simulink model "SP_OEL"  (R2023b)
settings: Solver=VariableStepAuto  StartTime=0.0  StopTime=1  RelTol=1e-3
undefined symbols (not defined in the file or in its folder): relay1, relay2, source
libraries: ee_lib x31, fl_lib x16, eeGeneralControl x8, nesl_utility x7, simulink x4, simulink_extras x4, spspowerguiLib x1
(part 2 of 2)

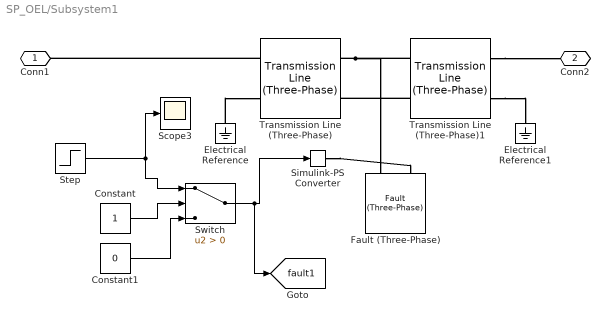
== system SP_OEL/Subsystem1 ==
  Constant : Constant
  Constant1 : Constant  Value=0
  Electrical Reference : fl_lib/Electrical/Electrical Elements/Electrical Reference
  Electrical Reference1 : fl_lib/Electrical/Electrical Elements/Electrical Reference
  Fault (Three-Phase) : ee_lib/Utilities/Fault (Three-Phase)  fault_type_option=1  R_pn_fault=1e-6 Ohm  R_ng_fault=1e-6 Ohm  exposemeasurement=ee.enum.exposemeasurement.hidden  enable_external_fault=ee.enum.external_fault.visible  fault_threshold=0.5  fault_condition=1  fault_resettable=1  enable_temporal_fault=0  fault_start_time=1 s  fault_duration=0.1 s  G_parasitic=1e-6 1/Ohm
      settings: InternalSimscapePortConfiguration="{\"Bottom\":[],\"Left\":[{\"id\":\"N\",\"label\":\"~\",\"type\":\"foundation.electrical.three_phase\"},{\"id\":\"F\",\"label\":\"F\",\"type\":\"input\"}],\"Right\":[],\"Top\":[]}"
  Scope3 : Scope
  Simulink-PS Converter : nesl_utility/Simulink-PS Converter  PhysicalDomain=network_engine_domain  SubClassName=ps_input  LeftPortType=input  RightPortType=output  PseudoPeriodic=off  Frequencies=[]  NoiseDistribution=none  NoiseParameters=[]  Unit=1  AffineConversion=off  FilteringAndDerivatives=provide  SimscapeFilterOrder=1  InputFilterTimeConstant=0.001  UdotUserProvided=0
  Step : Step  Time=0  After=0  SampleTime=0
  Switch : Switch  Criteria=u2 > Threshold  SaturateOnIntegerOverflow=off  InputSameDT=off
  Transmission Line (Three-Phase) : ee_lib/Passive/Lines/Transmission Line (Three-Phase)  length=1 km  freq=50 Hz  R=0.0268 Ohm/km  L=0.32 mH/km  M=0.0 mH/km  Cl=0.37 uF/km  Cg=0.1 uF/km  Rm=0 Ohm/km  ModelTwoSections=ee.enum.enable.no  N=1  InterfacePosition=0.5 km  N1sec=1  N2sec=1  Access_ground=ee.enum.enable.no  R_parasitic=1e-4 Ohm  G_parasitic=1e-4 1/Ohm  EnableFault=false  fault_type_option=ee.enum.fault_type_option.ag  R_pn_fault=1e-3 Ohm  R_ng_fault=1e-3 Ohm  unfaulted_G_parasitic=1e-6 1/Ohm
      settings: InternalSimscapePortConfiguration="{\"Bottom\":[],\"Left\":[{\"id\":\"N1\",\"label\":\"~1\",\"type\":\"foundation.electrical.three_phase\"},{\"id\":\"g1\",\"label\":\"g1\",\"type\":\"foundation.electrical.electrical\"}],\"Right\":[{\"id\":\"N2\",\"label\":\"~2\",\"type\":\"foundation.electrical.three_phase\"},{\"id\":\"g2\",\"label\":\"g2\",\"type\":\"foundation.electrical.electrical\"}],\"Top\":[]}"
  Transmission Line (Three-Phase)1 : ee_lib/Passive/Lines/Transmission Line (Three-Phase)  length=9 km  freq=50 Hz  R=0.0268 Ohm/km  L=0.32 mH/km  M=0.0 mH/km  Cl=0.37 uF/km  Cg=0.1 uF/km  Rm=0 Ohm/km  ModelTwoSections=ee.enum.enable.no  N=1  InterfacePosition=0.5 km  N1sec=1  N2sec=1  Access_ground=ee.enum.enable.no  R_parasitic=1e-4 Ohm  G_parasitic=1e-4 1/Ohm  EnableFault=false  fault_type_option=ee.enum.fault_type_option.ag  R_pn_fault=1e-3 Ohm  R_ng_fault=1e-3 Ohm  unfaulted_G_parasitic=1e-6 1/Ohm
      settings: InternalSimscapePortConfiguration="{\"Bottom\":[],\"Left\":[{\"id\":\"N1\",\"label\":\"~1\",\"type\":\"foundation.electrical.three_phase\"},{\"id\":\"g1\",\"label\":\"g1\",\"type\":\"foundation.electrical.electrical\"}],\"Right\":[{\"id\":\"N2\",\"label\":\"~2\",\"type\":\"foundation.electrical.three_phase\"},{\"id\":\"g2\",\"label\":\"g2\",\"type\":\"foundation.electrical.electrical\"}],\"Top\":[]}"
  Conn1 : PMIOPort  Side=Left
  Conn2 : PMIOPort  Port=2  Side=Right
  tag scope: fault1=global
  wires:
  Switch/1 -> [fault1], Simulink-PS Converter/1
  Constant1/1 -> Switch/3
  Constant/1 -> Switch/2
  Step/1 -> Scope3/1, Switch/1
  connections:
  Transmission Line (Three-Phase)1/RConn2 -- Electrical Reference1/LConn1
  Electrical Reference/LConn1 -- Transmission Line (Three-Phase)/LConn2
  Simulink-PS Converter/RConn1 -- Fault (Three-Phase)/LConn2
  Transmission Line (Three-Phase)1/RConn1 -- Conn2/RConn1
  Transmission Line (Three-Phase)/RConn1 -- Transmission Line (Three-Phase)1/LConn1 -- Fault (Three-Phase)/LConn1
  Transmission Line (Three-Phase)/LConn1 -- Conn1/RConn1
  Transmission Line (Three-Phase)1/LConn2 -- Transmission Line (Three-Phase)/RConn2

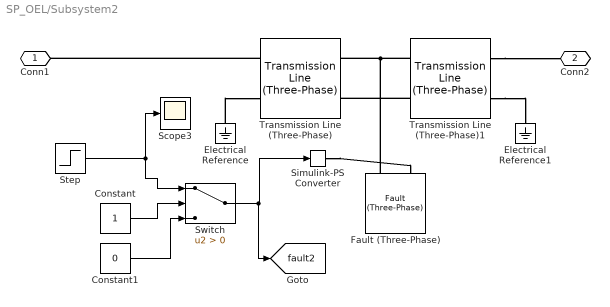
== system SP_OEL/Subsystem2 ==
  Constant : Constant
  Constant1 : Constant  Value=0
  Electrical Reference : fl_lib/Electrical/Electrical Elements/Electrical Reference
  Electrical Reference1 : fl_lib/Electrical/Electrical Elements/Electrical Reference
  Fault (Three-Phase) : ee_lib/Utilities/Fault (Three-Phase)  fault_type_option=1  R_pn_fault=1e-6 Ohm  R_ng_fault=1e-6 Ohm  exposemeasurement=ee.enum.exposemeasurement.hidden  enable_external_fault=ee.enum.external_fault.visible  fault_threshold=0.5  fault_condition=1  fault_resettable=1  enable_temporal_fault=0  fault_start_time=1 s  fault_duration=0.1 s  G_parasitic=1e-6 1/Ohm
      settings: InternalSimscapePortConfiguration="{\"Bottom\":[],\"Left\":[{\"id\":\"N\",\"label\":\"~\",\"type\":\"foundation.electrical.three_phase\"},{\"id\":\"F\",\"label\":\"F\",\"type\":\"input\"}],\"Right\":[],\"Top\":[]}"
  Scope3 : Scope
  Simulink-PS Converter : nesl_utility/Simulink-PS Converter  PhysicalDomain=network_engine_domain  SubClassName=ps_input  LeftPortType=input  RightPortType=output  PseudoPeriodic=off  Frequencies=[]  NoiseDistribution=none  NoiseParameters=[]  Unit=1  AffineConversion=off  FilteringAndDerivatives=provide  SimscapeFilterOrder=1  InputFilterTimeConstant=0.001  UdotUserProvided=0
  Step : Step  Time=0.2  SampleTime=0
  Switch : Switch  Criteria=u2 > Threshold  SaturateOnIntegerOverflow=off  InputSameDT=off
  Transmission Line (Three-Phase) : ee_lib/Passive/Lines/Transmission Line (Three-Phase)  length=1 km  freq=50 Hz  R=0.0268 Ohm/km  L=0.32 mH/km  M=0.0 mH/km  Cl=0.37 uF/km  Cg=0.1 uF/km  Rm=0 Ohm/km  ModelTwoSections=ee.enum.enable.no  N=1  InterfacePosition=0.5 km  N1sec=1  N2sec=1  Access_ground=ee.enum.enable.no  R_parasitic=1e-4 Ohm  G_parasitic=1e-4 1/Ohm  EnableFault=false  fault_type_option=ee.enum.fault_type_option.ag  R_pn_fault=1e-3 Ohm  R_ng_fault=1e-3 Ohm  unfaulted_G_parasitic=1e-6 1/Ohm
      settings: InternalSimscapePortConfiguration="{\"Bottom\":[],\"Left\":[{\"id\":\"N1\",\"label\":\"~1\",\"type\":\"foundation.electrical.three_phase\"},{\"id\":\"g1\",\"label\":\"g1\",\"type\":\"foundation.electrical.electrical\"}],\"Right\":[{\"id\":\"N2\",\"label\":\"~2\",\"type\":\"foundation.electrical.three_phase\"},{\"id\":\"g2\",\"label\":\"g2\",\"type\":\"foundation.electrical.electrical\"}],\"Top\":[]}"
  Transmission Line (Three-Phase)1 : ee_lib/Passive/Lines/Transmission Line (Three-Phase)  length=9 km  freq=50 Hz  R=0.0268 Ohm/km  L=0.32 mH/km  M=0.0 mH/km  Cl=0.37 uF/km  Cg=0.1 uF/km  Rm=0 Ohm/km  ModelTwoSections=ee.enum.enable.no  N=1  InterfacePosition=0.5 km  N1sec=1  N2sec=1  Access_ground=ee.enum.enable.no  R_parasitic=1e-4 Ohm  G_parasitic=1e-4 1/Ohm  EnableFault=false  fault_type_option=ee.enum.fault_type_option.ag  R_pn_fault=1e-3 Ohm  R_ng_fault=1e-3 Ohm  unfaulted_G_parasitic=1e-6 1/Ohm
      settings: InternalSimscapePortConfiguration="{\"Bottom\":[],\"Left\":[{\"id\":\"N1\",\"label\":\"~1\",\"type\":\"foundation.electrical.three_phase\"},{\"id\":\"g1\",\"label\":\"g1\",\"type\":\"foundation.electrical.electrical\"}],\"Right\":[{\"id\":\"N2\",\"label\":\"~2\",\"type\":\"foundation.electrical.three_phase\"},{\"id\":\"g2\",\"label\":\"g2\",\"type\":\"foundation.electrical.electrical\"}],\"Top\":[]}"
  Conn1 : PMIOPort  Side=Left
  Conn2 : PMIOPort  Port=2  Side=Right
  tag scope: fault2=global
  wires:
  Step/1 -> Switch/1, Scope3/1
  Constant/1 -> Switch/2
  Constant1/1 -> Switch/3
  Switch/1 -> [fault2], Simulink-PS Converter/1
  connections:
  Transmission Line (Three-Phase)1/LConn2 -- Transmission Line (Three-Phase)/RConn2
  Transmission Line (Three-Phase)/LConn1 -- Conn1/RConn1
  Transmission Line (Three-Phase)1/LConn1 -- Fault (Three-Phase)/LConn1 -- Transmission Line (Three-Phase)/RConn1
  Transmission Line (Three-Phase)1/RConn1 -- Conn2/RConn1
  Simulink-PS Converter/RConn1 -- Fault (Three-Phase)/LConn2
  Electrical Reference/LConn1 -- Transmission Line (Three-Phase)/LConn2
  Transmission Line (Three-Phase)1/RConn2 -- Electrical Reference1/LConn1

== system SP_OEL/ Sensor1/Sensor dynamics ==
  V : Inport
  Demux : Demux  Outputs=3
  Mux : Mux  Inputs=3
  Transfer Fcn : TransferFcn  Denominator=[relay1.sampleTime 1]
  Transfer Fcn1 : TransferFcn  Denominator=[relay1.sampleTime 1]
  Transfer Fcn2 : TransferFcn  Denominator=[relay1.sampleTime 1]
  I : Outport
  wires:
  Transfer Fcn/1 -> Mux/1
  Demux/1 -> Transfer Fcn/1
  Demux/3 -> Transfer Fcn2/1
  Mux/1 -> I/1
  Transfer Fcn2/1 -> Mux/3
  Transfer Fcn1/1 -> Mux/2
  Demux/2 -> Transfer Fcn1/1
  V/1 -> Demux/1

== system SP_OEL/ Sensor2/Sensor dynamics ==
  V : Inport
  Demux : Demux  Outputs=3
  Mux : Mux  Inputs=3
  Transfer Fcn : TransferFcn  Denominator=[relay2.sampleTime 1]
  Transfer Fcn1 : TransferFcn  Denominator=[relay2.sampleTime 1]
  Transfer Fcn2 : TransferFcn  Denominator=[relay2.sampleTime 1]
  I : Outport
  wires:
  Transfer Fcn/1 -> Mux/1
  Demux/1 -> Transfer Fcn/1
  Demux/3 -> Transfer Fcn2/1
  Mux/1 -> I/1
  Transfer Fcn2/1 -> Mux/3
  Transfer Fcn1/1 -> Mux/2
  Demux/2 -> Transfer Fcn1/1
  V/1 -> Demux/1

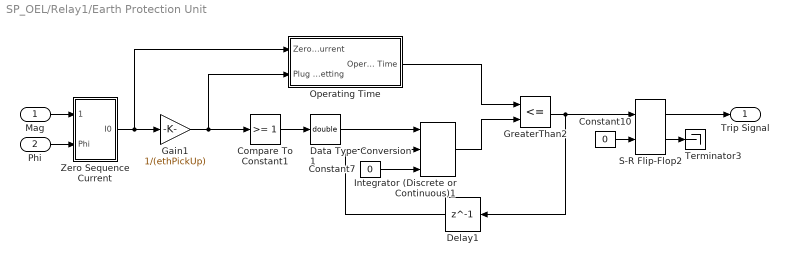
== system SP_OEL/Relay1/Earth Protection Unit ==
  Mag : Inport
  Phi : Inport  Port=2
  Compare To Constant1 : simulink/Logic and Bit Operations/Compare To Constant  relop=>=  const=1  OutDataTypeStr=boolean
  Constant10 : Constant  Value=0  OutDataTypeStr=boolean
  Constant7 : Constant  Value=0  OutDataTypeStr=double
  Data Type Conversion1 : DataTypeConversion  OutDataTypeStr=double  SaturateOnIntegerOverflow=off  RndMeth=Floor
  Delay1 : Delay  DelayLength=1
  Gain1 : Gain  Gain=1/(ethPickUp)
  GreaterThan2 : RelationalOperator  Operator=<=  OutDataTypeStr=boolean  RndMeth=Simplest  InputSameDT=off
  Integrator (Discrete or Continuous)1 : eeGeneralControl/Integrator (Discrete or Continuous)  LabelModeActiveChoice=Discrete  ExternalReset=falling  LimitType=Anti-windup  B=inf  A=-inf  Ts=sampleTime
  Operating Time : Subsystem
  S-R Flip-Flop2 : simulink_extras/Flip Flops/S-R Flip-Flop  initial_condition=0
  Terminator3 : Terminator
  Zero Sequence Current : Subsystem
  Trip Signal : Outport
  wires:
  Gain1/1 -> Operating Time/2(Plug Setting), Compare To Constant1/1
  Compare To Constant1/1 -> Data Type Conversion1/1
  GreaterThan2/1 -> Delay1/1, S-R Flip-Flop2/1
  Delay1/1 -> Integrator (Discrete or Continuous)1/2
  Constant10/1 -> S-R Flip-Flop2/2
  Zero Sequence Current/1(I0) -> Gain1/1, Operating Time/1(Zero Sequence Current)
  Data Type Conversion1/1 -> Integrator (Discrete or Continuous)1/1
  Integrator (Discrete or Continuous)1/1 -> GreaterThan2/2
  Operating Time/1(Operating Time) -> GreaterThan2/1
  S-R Flip-Flop2/2 -> Terminator3/1
  Constant7/1 -> Integrator (Discrete or Continuous)1/3
  Phi/1 -> Zero Sequence Current/2(Phi)
  Mag/1 -> Zero Sequence Current/1(Mag)
  S-R Flip-Flop2/1 -> Trip Signal/1

== system SP_OEL/Relay1/Fourier Analysis ==
  Current : Inport
  Add1 : Sum  Inputs=-+
  Delay3 : Delay  DelayLength=1
  Fourier Analysis2 : eeGeneralControl/Fourier Analysis  f=ratedFrequency  n=[1]  M0=0  Ph0=0  BufferSize=8192  Ts=sampleTime
  Gain : Gain  Gain=1/sqrt(2)
  Moving Average : eeGeneralControl/Moving Average  VariantControl=Variant1  LabelModeActiveChoice=Discrete  f=50  x0=0  BufferSize=8192  Ts=sampleTime
  Magnitude : Outport
  Angle : Outport  Port=2
  wires:
  Delay3/1 -> Add1/2, Moving Average/1
  Current/1 -> Delay3/1
  Fourier Analysis2/2 -> Angle/1
  Moving Average/1 -> Add1/1
  Add1/1 -> Fourier Analysis2/1
  Fourier Analysis2/1 -> Gain/1
  Gain/1 -> Magnitude/1

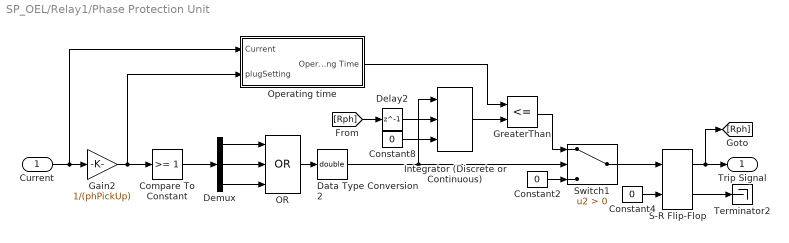
== system SP_OEL/Relay1/Phase Protection Unit ==
  Current : Inport
  Compare To Constant : simulink/Logic and Bit Operations/Compare To Constant  relop=>=  const=1  OutDataTypeStr=boolean
  Constant2 : Constant  Value=0  OutDataTypeStr=boolean
  Constant4 : Constant  Value=0  OutDataTypeStr=boolean
  Constant8 : Constant  Value=0  OutDataTypeStr=double
  Data Type Conversion2 : DataTypeConversion  OutDataTypeStr=double  SaturateOnIntegerOverflow=off  RndMeth=Floor
  Delay2 : Delay  DelayLength=1
  Demux : Demux  Outputs=3
  Gain2 : Gain  Gain=1/(phPickUp)
  GreaterThan : RelationalOperator  Operator=<=  OutDataTypeStr=boolean  RndMeth=Simplest  InputSameDT=off
  Integrator (Discrete or Continuous) : eeGeneralControl/Integrator (Discrete or Continuous)  LabelModeActiveChoice=Discrete  ExternalReset=falling  LimitType=Anti-windup  B=inf  A=-inf  Ts=sampleTime
  OR : Logic  Operator=OR  Inputs=3  IconShape=distinctive  AllPortsSameDT=off  OutDataTypeStr=boolean
  "Operating time " : Subsystem
  S-R Flip-Flop : simulink_extras/Flip Flops/S-R Flip-Flop  initial_condition=0
  Switch1 : Switch  Criteria=u2 > Threshold  OutDataTypeStr=boolean  SaturateOnIntegerOverflow=off  InputSameDT=off
  Terminator2 : Terminator
  Trip Signal : Outport
  wires:
  Data Type Conversion2/1 -> Integrator (Discrete or Continuous)/1, Switch1/2
  Gain2/1 -> "Operating time "/2(plugSetting), Compare To Constant/1
  Constant2/1 -> Switch1/3
  Demux/2 -> OR/2
  OR/1 -> Data Type Conversion2/1
  Integrator (Discrete or Continuous)/1 -> GreaterThan/2
  Demux/3 -> OR/3
  Current/1 -> Gain2/1, "Operating time "/1(Current)
  GreaterThan/1 -> Switch1/1
  "Operating time "/1(Operating Time) -> GreaterThan/1
  Constant4/1 -> S-R Flip-Flop/2
  S-R Flip-Flop/2 -> Terminator2/1
  Switch1/1 -> S-R Flip-Flop/1
  Demux/1 -> OR/1
  Constant8/1 -> Integrator (Discrete or Continuous)/3
  Compare To Constant/1 -> Demux/1
  S-R Flip-Flop/1 -> Trip Signal/1, [Rph]
  Delay2/1 -> Integrator (Discrete or Continuous)/2
  [Rph] -> Delay2/1

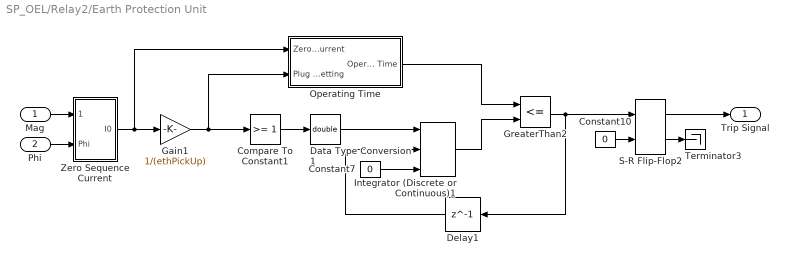
== system SP_OEL/Relay2/Earth Protection Unit ==
  Mag : Inport
  Phi : Inport  Port=2
  Compare To Constant1 : simulink/Logic and Bit Operations/Compare To Constant  relop=>=  const=1  OutDataTypeStr=boolean
  Constant10 : Constant  Value=0  OutDataTypeStr=boolean
  Constant7 : Constant  Value=0  OutDataTypeStr=double
  Data Type Conversion1 : DataTypeConversion  OutDataTypeStr=double  SaturateOnIntegerOverflow=off  RndMeth=Floor
  Delay1 : Delay  DelayLength=1
  Gain1 : Gain  Gain=1/(ethPickUp)
  GreaterThan2 : RelationalOperator  Operator=<=  OutDataTypeStr=boolean  RndMeth=Simplest  InputSameDT=off
  Integrator (Discrete or Continuous)1 : eeGeneralControl/Integrator (Discrete or Continuous)  LabelModeActiveChoice=Discrete  ExternalReset=falling  LimitType=Anti-windup  B=inf  A=-inf  Ts=sampleTime
  Operating Time : Subsystem
  S-R Flip-Flop2 : simulink_extras/Flip Flops/S-R Flip-Flop  initial_condition=0
  Terminator3 : Terminator
  Zero Sequence Current : Subsystem
  Trip Signal : Outport
  wires:
  Gain1/1 -> Operating Time/2(Plug Setting), Compare To Constant1/1
  Compare To Constant1/1 -> Data Type Conversion1/1
  GreaterThan2/1 -> Delay1/1, S-R Flip-Flop2/1
  Delay1/1 -> Integrator (Discrete or Continuous)1/2
  Constant10/1 -> S-R Flip-Flop2/2
  Zero Sequence Current/1(I0) -> Gain1/1, Operating Time/1(Zero Sequence Current)
  Data Type Conversion1/1 -> Integrator (Discrete or Continuous)1/1
  Integrator (Discrete or Continuous)1/1 -> GreaterThan2/2
  Operating Time/1(Operating Time) -> GreaterThan2/1
  S-R Flip-Flop2/2 -> Terminator3/1
  Constant7/1 -> Integrator (Discrete or Continuous)1/3
  Phi/1 -> Zero Sequence Current/2(Phi)
  Mag/1 -> Zero Sequence Current/1(Mag)
  S-R Flip-Flop2/1 -> Trip Signal/1

== system SP_OEL/Relay2/Fourier Analysis ==
  Current : Inport
  Add1 : Sum  Inputs=-+
  Delay3 : Delay  DelayLength=1
  Fourier Analysis2 : eeGeneralControl/Fourier Analysis  f=ratedFrequency  n=[1]  M0=0  Ph0=0  BufferSize=8192  Ts=sampleTime
  Gain : Gain  Gain=1/sqrt(2)
  Moving Average : eeGeneralControl/Moving Average  VariantControl=Variant1  LabelModeActiveChoice=Discrete  f=50  x0=0  BufferSize=8192  Ts=sampleTime
  Magnitude : Outport
  Angle : Outport  Port=2
  wires:
  Delay3/1 -> Add1/2, Moving Average/1
  Current/1 -> Delay3/1
  Fourier Analysis2/2 -> Angle/1
  Moving Average/1 -> Add1/1
  Add1/1 -> Fourier Analysis2/1
  Fourier Analysis2/1 -> Gain/1
  Gain/1 -> Magnitude/1

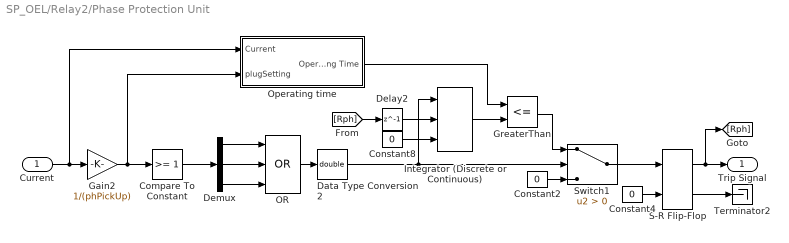
== system SP_OEL/Relay2/Phase Protection Unit ==
  Current : Inport
  Compare To Constant : simulink/Logic and Bit Operations/Compare To Constant  relop=>=  const=1  OutDataTypeStr=boolean
  Constant2 : Constant  Value=0  OutDataTypeStr=boolean
  Constant4 : Constant  Value=0  OutDataTypeStr=boolean
  Constant8 : Constant  Value=0  OutDataTypeStr=double
  Data Type Conversion2 : DataTypeConversion  OutDataTypeStr=double  SaturateOnIntegerOverflow=off  RndMeth=Floor
  Delay2 : Delay  DelayLength=1
  Demux : Demux  Outputs=3
  Gain2 : Gain  Gain=1/(phPickUp)
  GreaterThan : RelationalOperator  Operator=<=  OutDataTypeStr=boolean  RndMeth=Simplest  InputSameDT=off
  Integrator (Discrete or Continuous) : eeGeneralControl/Integrator (Discrete or Continuous)  LabelModeActiveChoice=Discrete  ExternalReset=falling  LimitType=Anti-windup  B=inf  A=-inf  Ts=sampleTime
  OR : Logic  Operator=OR  Inputs=3  IconShape=distinctive  AllPortsSameDT=off  OutDataTypeStr=boolean
  "Operating time " : Subsystem
  S-R Flip-Flop : simulink_extras/Flip Flops/S-R Flip-Flop  initial_condition=0
  Switch1 : Switch  Criteria=u2 > Threshold  OutDataTypeStr=boolean  SaturateOnIntegerOverflow=off  InputSameDT=off
  Terminator2 : Terminator
  Trip Signal : Outport
  wires:
  Data Type Conversion2/1 -> Integrator (Discrete or Continuous)/1, Switch1/2
  Gain2/1 -> "Operating time "/2(plugSetting), Compare To Constant/1
  Constant2/1 -> Switch1/3
  Demux/2 -> OR/2
  OR/1 -> Data Type Conversion2/1
  Integrator (Discrete or Continuous)/1 -> GreaterThan/2
  Demux/3 -> OR/3
  Current/1 -> Gain2/1, "Operating time "/1(Current)
  GreaterThan/1 -> Switch1/1
  "Operating time "/1(Operating Time) -> GreaterThan/1
  Constant4/1 -> S-R Flip-Flop/2
  S-R Flip-Flop/2 -> Terminator2/1
  Switch1/1 -> S-R Flip-Flop/1
  Demux/1 -> OR/1
  Constant8/1 -> Integrator (Discrete or Continuous)/3
  Compare To Constant/1 -> Demux/1
  S-R Flip-Flop/1 -> Trip Signal/1, [Rph]
  Delay2/1 -> Integrator (Discrete or Continuous)/2
  [Rph] -> Delay2/1

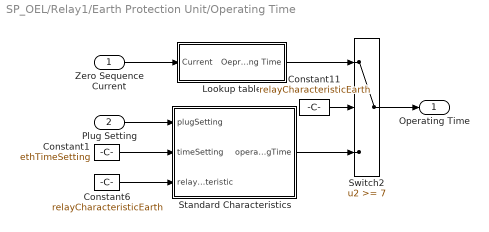
== system SP_OEL/Relay1/Earth Protection Unit/Operating Time ==
  Zero Sequence Current : Inport
  Plug Setting : Inport  Port=2
  Constant1 : Constant  Value=ethTimeSetting
  Constant11 : Constant  Value=relayCharacteristicEarth
  Constant6 : Constant  Value=relayCharacteristicEarth
  Lookup table : Subsystem
  Standard Characteristics : MATLAB Function  TreatAsAtomicUnit=on
  Switch2 : Switch  Threshold=7  SaturateOnIntegerOverflow=off  InputSameDT=off
  Operating Time : Outport
  wires:
  Constant1/1 -> Standard Characteristics/2(timeSetting)
  Lookup table/1(Oeprating Time) -> Switch2/1
  Constant6/1 -> Standard Characteristics/3(relayCharacteristic)
  Plug Setting/1 -> Standard Characteristics/1(plugSetting)
  Standard Characteristics/1(operatingTime) -> Switch2/3
  Constant11/1 -> Switch2/2
  Switch2/1 -> Operating Time/1
  Zero Sequence Current/1 -> Lookup table/1(Current)

== system SP_OEL/Relay1/Earth Protection Unit/Zero Sequence Current ==
  Mag : Inport
  Phi : Inport  Port=2
  Add : Sum  Inputs=+++
  Complex to Magnitude-Angle : ComplexToMagnitudeAngle  Output=Magnitude
  Demux1 : Demux  Outputs=3
  Gain : Gain  Gain=1/3
  Magnitude-Angle to Complex : MagnitudeAngleToComplex
  I0 : Outport
  wires:
  Demux1/2 -> Add/2
  Demux1/3 -> Add/3
  Phi/1 -> Magnitude-Angle to Complex/2
  Complex to Magnitude-Angle/1 -> Gain/1
  Demux1/1 -> Add/1
  Mag/1 -> Magnitude-Angle to Complex/1
  Magnitude-Angle to Complex/1 -> Demux1/1
  Add/1 -> Complex to Magnitude-Angle/1
  Gain/1 -> I0/1

== system SP_OEL/Relay1/Phase Protection Unit/Operating time  ==
  Current : Inport
  plugSetting : Inport  Port=2
  Constant : Constant  Value=phTimeSetting  VectorParams1D=off
  Constant3 : Constant  Value=relayCharacteristicPhase
  Constant9 : Constant  Value=relayCharacteristicPhase
  "Lookup table " : Subsystem
  MATLAB Function : MATLAB Function  TreatAsAtomicUnit=on
  Switch : Switch  Threshold=7  SaturateOnIntegerOverflow=off  InputSameDT=off
  Operating Time : Outport
  wires:
  Switch/1 -> Operating Time/1
  plugSetting/1 -> MATLAB Function/1(plugSetting)
  Constant9/1 -> Switch/2
  Constant/1 -> MATLAB Function/2(timeSetting)
  Constant3/1 -> MATLAB Function/3(relayCharacteristic)
  MATLAB Function/1(operatingTime) -> Switch/3
  "Lookup table "/1(Operating Time) -> Switch/1
  Current/1 -> "Lookup table "/1(Current)

== system SP_OEL/Relay2/Earth Protection Unit/Operating Time ==
  Zero Sequence Current : Inport
  Plug Setting : Inport  Port=2
  Constant1 : Constant  Value=ethTimeSetting
  Constant11 : Constant  Value=relayCharacteristicEarth
  Constant6 : Constant  Value=relayCharacteristicEarth
  Lookup table : Subsystem
  Standard Characteristics : MATLAB Function  TreatAsAtomicUnit=on
  Switch2 : Switch  Threshold=7  SaturateOnIntegerOverflow=off  InputSameDT=off
  Operating Time : Outport
  wires:
  Constant1/1 -> Standard Characteristics/2(timeSetting)
  Lookup table/1(Oeprating Time) -> Switch2/1
  Constant6/1 -> Standard Characteristics/3(relayCharacteristic)
  Plug Setting/1 -> Standard Characteristics/1(plugSetting)
  Standard Characteristics/1(operatingTime) -> Switch2/3
  Constant11/1 -> Switch2/2
  Switch2/1 -> Operating Time/1
  Zero Sequence Current/1 -> Lookup table/1(Current)

== system SP_OEL/Relay2/Earth Protection Unit/Zero Sequence Current ==
  Mag : Inport
  Phi : Inport  Port=2
  Add : Sum  Inputs=+++
  Complex to Magnitude-Angle : ComplexToMagnitudeAngle  Output=Magnitude
  Demux1 : Demux  Outputs=3
  Gain : Gain  Gain=1/3
  Magnitude-Angle to Complex : MagnitudeAngleToComplex
  I0 : Outport
  wires:
  Demux1/2 -> Add/2
  Demux1/3 -> Add/3
  Phi/1 -> Magnitude-Angle to Complex/2
  Complex to Magnitude-Angle/1 -> Gain/1
  Demux1/1 -> Add/1
  Mag/1 -> Magnitude-Angle to Complex/1
  Magnitude-Angle to Complex/1 -> Demux1/1
  Add/1 -> Complex to Magnitude-Angle/1
  Gain/1 -> I0/1

== system SP_OEL/Relay2/Phase Protection Unit/Operating time  ==
  Current : Inport
  plugSetting : Inport  Port=2
  Constant : Constant  Value=phTimeSetting  VectorParams1D=off
  Constant3 : Constant  Value=relayCharacteristicPhase
  Constant9 : Constant  Value=relayCharacteristicPhase
  "Lookup table " : Subsystem
  MATLAB Function : MATLAB Function  TreatAsAtomicUnit=on
  Switch : Switch  Threshold=7  SaturateOnIntegerOverflow=off  InputSameDT=off
  Operating Time : Outport
  wires:
  Switch/1 -> Operating Time/1
  plugSetting/1 -> MATLAB Function/1(plugSetting)
  Constant9/1 -> Switch/2
  Constant/1 -> MATLAB Function/2(timeSetting)
  Constant3/1 -> MATLAB Function/3(relayCharacteristic)
  MATLAB Function/1(operatingTime) -> Switch/3
  "Lookup table "/1(Operating Time) -> Switch/1
  Current/1 -> "Lookup table "/1(Current)

== system SP_OEL/Relay1/Earth Protection Unit/Operating Time/Lookup table ==
  Current : Inport
  2-D Lookup Table1 : Lookup_n-D  BreakpointsForDimension1=currentEarth  BreakpointsForDimension2=tmsEarth  Table=topEarth  InterpMethod=Cubic spline  ExtrapMethod=Cubic spline  InternalRulePriority=Speed  RndMeth=Simplest
      settings: InputPortMap=u0,u1
  Constant13 : Constant  Value=ethTimeSetting
  Constant16 : Constant  Value=topEarthActual
  Constant17 : Constant  Value=relayCharacteristicEarth
  Switch4 : Switch  Threshold=8  SaturateOnIntegerOverflow=off  InputSameDT=off
  Oeprating Time : Outport
  wires:
  Current/1 -> 2-D Lookup Table1/1
  Constant17/1 -> Switch4/2
  2-D Lookup Table1/1 -> Switch4/1
  Constant16/1 -> Switch4/3
  Constant13/1 -> 2-D Lookup Table1/2
  Switch4/1 -> Oeprating Time/1

== system SP_OEL/Relay1/Phase Protection Unit/Operating time /Lookup table  ==
  Current : Inport
  2-D Lookup Table : Lookup_n-D  BreakpointsForDimension1=currentPhase  BreakpointsForDimension2=tmsPhase  Table=topPhase  InterpMethod=Cubic spline  ExtrapMethod=Cubic spline  InternalRulePriority=Speed  RndMeth=Simplest
      settings: InputPortMap=u0,u1
  Constant12 : Constant  Value=phTimeSetting  VectorParams1D=off
  Constant14 : Constant  Value=topPhaseActual
  Constant15 : Constant  Value=relayCharacteristicPhase
  Demux2 : Demux  Outputs=3
  Max : MinMax  Function=max  Inputs=3
  Switch3 : Switch  Threshold=8  SaturateOnIntegerOverflow=off  InputSameDT=off
  Operating Time : Outport
  wires:
  Constant15/1 -> Switch3/2
  Current/1 -> Demux2/1
  Constant12/1 -> 2-D Lookup Table/2
  Demux2/2 -> Max/2
  Demux2/1 -> Max/1
  Constant14/1 -> Switch3/3
  2-D Lookup Table/1 -> Switch3/1
  Demux2/3 -> Max/3
  Switch3/1 -> Operating Time/1
  Max/1 -> 2-D Lookup Table/1

== system SP_OEL/Relay2/Earth Protection Unit/Operating Time/Lookup table ==
  Current : Inport
  2-D Lookup Table1 : Lookup_n-D  BreakpointsForDimension1=currentEarth  BreakpointsForDimension2=tmsEarth  Table=topEarth  InterpMethod=Cubic spline  ExtrapMethod=Cubic spline  InternalRulePriority=Speed  RndMeth=Simplest
      settings: InputPortMap=u0,u1
  Constant13 : Constant  Value=ethTimeSetting
  Constant16 : Constant  Value=topEarthActual
  Constant17 : Constant  Value=relayCharacteristicEarth
  Switch4 : Switch  Threshold=8  SaturateOnIntegerOverflow=off  InputSameDT=off
  Oeprating Time : Outport
  wires:
  Current/1 -> 2-D Lookup Table1/1
  Constant17/1 -> Switch4/2
  2-D Lookup Table1/1 -> Switch4/1
  Constant16/1 -> Switch4/3
  Constant13/1 -> 2-D Lookup Table1/2
  Switch4/1 -> Oeprating Time/1

== system SP_OEL/Relay2/Phase Protection Unit/Operating time /Lookup table  ==
  Current : Inport
  2-D Lookup Table : Lookup_n-D  BreakpointsForDimension1=currentPhase  BreakpointsForDimension2=tmsPhase  Table=topPhase  InterpMethod=Cubic spline  ExtrapMethod=Cubic spline  InternalRulePriority=Speed  RndMeth=Simplest
      settings: InputPortMap=u0,u1
  Constant12 : Constant  Value=phTimeSetting  VectorParams1D=off
  Constant14 : Constant  Value=topPhaseActual
  Constant15 : Constant  Value=relayCharacteristicPhase
  Demux2 : Demux  Outputs=3
  Max : MinMax  Function=max  Inputs=3
  Switch3 : Switch  Threshold=8  SaturateOnIntegerOverflow=off  InputSameDT=off
  Operating Time : Outport
  wires:
  Constant15/1 -> Switch3/2
  Current/1 -> Demux2/1
  Constant12/1 -> 2-D Lookup Table/2
  Demux2/2 -> Max/2
  Demux2/1 -> Max/1
  Constant14/1 -> Switch3/3
  2-D Lookup Table/1 -> Switch3/1
  Demux2/3 -> Max/3
  Switch3/1 -> Operating Time/1
  Max/1 -> 2-D Lookup Table/1

== matlab function SP_OEL/Relay2/Earth Protection Unit/Operating Time/Standard Characteristics ==
  data: plugSetting input; operatingTime output; timeSetting input; relayCharacteristic input
function operatingTime = fcn(plugSetting,timeSetting,relayCharacteristic)
   if plugSetting>1             % Fault condition
    switch relayCharacteristic  % Selection of relay characteristic
        case 1                  % IEC Normal Inverse
          a=0.14;      
          b=0.02;
          c=0;
        case 2                  % IEC Very Inverse
           a=13.5;
           b=1;
           c=0;
        case 3                  % IEC Extremely Inverse
            a=80;
            b=2;
            c=0;
        case 4                  % IEC Moderately Inverse
            a=0.0515;
            b=0.02;
            c=0.114;
        case 5                  % IEEE Very Inverse
            a=19.61;
            b=2;
            c=0.491;
        case 6                  % IEEE Exteremely Inverse
            a=28.2;
            b=2;
            c=0.1217;
        otherwise               % Definite Time
            a=1;
            b=1;
            c=0;
            plugSetting=2;
    end               
         operatingTime=timeSetting*(a/(power(max(plugSetting),b)-1)+c);  % Calculate the oeprating time of the relay    
   else
       operatingTime=inf;  % Set relay operating time to infinite if there is no fault
   end
end

== matlab function SP_OEL/Relay2/Phase Protection Unit/Operating time /MATLAB Function ==
  data: plugSetting input; operatingTime output; timeSetting input; relayCharacteristic input
function operatingTime = fcn(plugSetting,timeSetting,relayCharacteristic)
   if plugSetting(1)>1 || plugSetting(2)>1 || plugSetting(3)>1  % Fault condition
    switch relayCharacteristic  % Selection of relay characteristic
        case 1                  % IEC Normal Inverse
          a=0.14;      
          b=0.02;
          c=0;
        case 2                  % IEC Very Inverse
           a=13.5;
           b=1;
           c=0;
        case 3                  % IEC Extremely Inverse
            a=80;
            b=2;
            c=0;
        case 4                  % IEC Moderately Inverse
            a=0.0515;
            b=0.02;
            c=0.114;
        case 5                  % IEEE Very Inverse
            a=19.61;
            b=2;
            c=0.491;
        case 6                  % IEEE Exteremely Inverse
            a=28.2;
            b=2;
            c=0.1217;
        otherwise               % Definite Time
            a=1;
            b=1;
            c=0;
            plugSetting=ones(3,1)*2;
    end           
         
         operatingTime=timeSetting*(a/(power(max(plugSetting),b)-1)+c);  % Calculate oeprating time of the relay  
   else
         operatingTime=inf;  % Set relay operating time to infinite if there is no fault
   end
end

== matlab function SP_OEL/Relay1/Earth Protection Unit/Operating Time/Standard Characteristics ==
  data: plugSetting input; operatingTime output; timeSetting input; relayCharacteristic input
function operatingTime = fcn(plugSetting,timeSetting,relayCharacteristic)
   if plugSetting>1             % Fault condition
    switch relayCharacteristic  % Selection of relay characteristic
        case 1                  % IEC Normal Inverse
          a=0.14;      
          b=0.02;
          c=0;
        case 2                  % IEC Very Inverse
           a=13.5;
           b=1;
           c=0;
        case 3                  % IEC Extremely Inverse
            a=80;
            b=2;
            c=0;
        case 4                  % IEC Moderately Inverse
            a=0.0515;
            b=0.02;
            c=0.114;
        case 5                  % IEEE Very Inverse
            a=19.61;
            b=2;
            c=0.491;
        case 6                  % IEEE Exteremely Inverse
            a=28.2;
            b=2;
            c=0.1217;
        otherwise               % Definite Time
            a=1;
            b=1;
            c=0;
            plugSetting=2;
    end               
         operatingTime=timeSetting*(a/(power(max(plugSetting),b)-1)+c);  % Calculate the oeprating time of the relay    
   else
       operatingTime=inf;  % Set relay operating time to infinite if there is no fault
   end
end

== matlab function SP_OEL/Relay1/Phase Protection Unit/Operating time /MATLAB Function ==
  data: plugSetting input; operatingTime output; timeSetting input; relayCharacteristic input
function operatingTime = fcn(plugSetting,timeSetting,relayCharacteristic)
   if plugSetting(1)>1 || plugSetting(2)>1 || plugSetting(3)>1  % Fault condition
    switch relayCharacteristic  % Selection of relay characteristic
        case 1                  % IEC Normal Inverse
          a=0.14;      
          b=0.02;
          c=0;
        case 2                  % IEC Very Inverse
           a=13.5;
           b=1;
           c=0;
        case 3                  % IEC Extremely Inverse
            a=80;
            b=2;
            c=0;
        case 4                  % IEC Moderately Inverse
            a=0.0515;
            b=0.02;
            c=0.114;
        case 5                  % IEEE Very Inverse
            a=19.61;
            b=2;
            c=0.491;
        case 6                  % IEEE Exteremely Inverse
            a=28.2;
            b=2;
            c=0.1217;
        otherwise               % Definite Time
            a=1;
            b=1;
            c=0;
            plugSetting=ones(3,1)*2;
    end           
         
         operatingTime=timeSetting*(a/(power(max(plugSetting),b)-1)+c);  % Calculate oeprating time of the relay  
   else
         operatingTime=inf;  % Set relay operating time to infinite if there is no fault
   end
end
